simulink model "cd2moscillator"  (R2016a)
settings: Solver=VariableStepAuto  StartTime=0.0  StopTime=10.0  FixedStep=0.07  MaxStep=0.038  RelTol=1e-3
values from neighbouring files (symbols this model uses):
  c1 = 120    [cd2massosc.m]
  c2 = 120    [cd2massosc.m]
  d1 = 0.5    [cd2massosc.m]
  d2 = 0.5    [cd2massosc.m]
  F = 100    [cd2massosc.m]
  g = 9.81    [cd2massosc.m]
  m1 = 4    [cd2massosc.m]
  m2 = 1    [cd2massosc.m]
  omega = 9.2    [cd2massosc.m]
  x10 = 0    [cd2massosc.m]
  x20 = 0    [cd2massosc.m]
settings Model: Creator=NachtHemdGangsta  LastModifiedBy=NachtHemd
settings DataIOCC: LimitDataPoints=on
settings DebuggingCC: AllowSymbolicDim=off
settings ModelReferenceCC: PropagateSignalLabelsOutOfModel=off
settings GRTTargetCC: GeneratePreprocessorConditionals=Use local settings

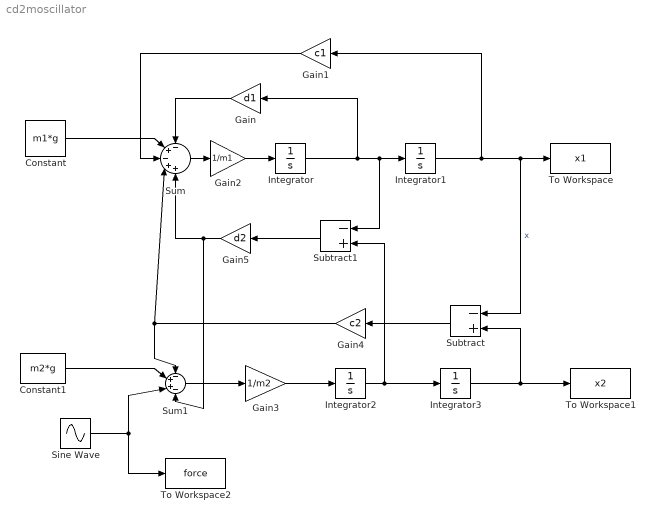
== system cd2moscillator ==
  Constant : Constant  Value=m1*g
  Constant1 : Constant  Value=m2*g
  Gain : Gain  Gain=d1
  Gain1 : Gain  Gain=c1
  Gain2 : Gain  Gain=1/m1
  Gain3 : Gain  Gain=1/m2
  Gain4 : Gain  Gain=c2
  Gain5 : Gain  Gain=d2
  Integrator : Integrator
  Integrator1 : Integrator  InitialCondition=x10
  Integrator2 : Integrator
  Integrator3 : Integrator  InitialCondition=x20
  Sine Wave : Sin  Amplitude=F  Frequency=omega  Phase=pi/2  SampleTime=0
  Subtract : Sum  Inputs=-+
  Subtract1 : Sum  Inputs=-+
  Sum : Sum  Inputs=-+-++
  Sum1 : Sum  Inputs=-++-
  To Workspace : ToWorkspace  VariableName=x1  SaveFormat=Structure With Time  SampleTime=-1
  To Workspace1 : ToWorkspace  VariableName=x2  SaveFormat=Structure With Time  SampleTime=-1
  To Workspace2 : ToWorkspace  VariableName=force  SaveFormat=Structure With Time  SampleTime=-1
  wires:
  Sum/1 -> Gain2/1
  Integrator1/1 -> Subtract/1, To Workspace/1, Gain1/1  "x"
  Integrator/1 -> Gain/1, Subtract1/1, Integrator1/1
  Gain/1 -> Sum/1
  Gain1/1 -> Sum/3
  Gain2/1 -> Integrator/1
  Sum1/1 -> Gain3/1
  Gain3/1 -> Integrator2/1
  Integrator2/1 -> Subtract1/2, Integrator3/1
  Constant/1 -> Sum/2
  Subtract/1 -> Gain4/1
  Gain4/1 -> Sum/4, Sum1/1
  Subtract1/1 -> Gain5/1
  Gain5/1 -> Sum1/4, Sum/5
  Constant1/1 -> Sum1/2
  Integrator3/1 -> Subtract/2, To Workspace1/1
  Sine Wave/1 -> Sum1/3, To Workspace2/1
